simulink model "S1File_JL2005MM"  (R2017a)
settings: Solver=VariableStepAuto  StartTime=0.0  StopTime=96  RelTol=1e-3
libraries: cstblocks x2
settings Model: Creator=ac8227  LastModifiedBy=ac8227

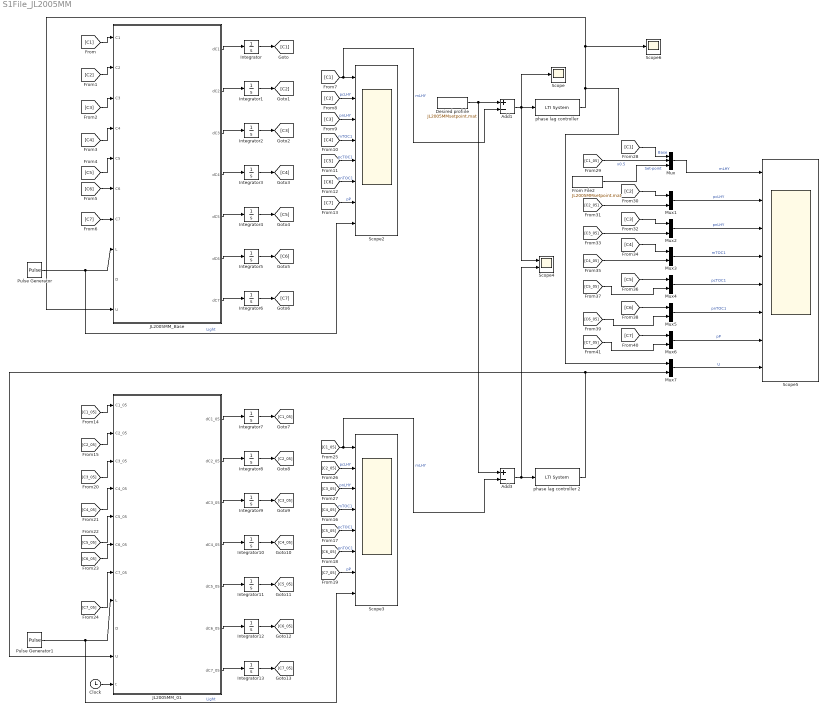
== system S1File_JL2005MM ==
  Add1 : Sum  Inputs=+-
  Add3 : Sum  Inputs=+-
  Clock : Clock
  Desired profiile : FromFile  FileName=JL2005MMsetpoint.mat  SampleTime=0
  From File2 : FromFile  FileName=JL2005MMsetpoint.mat  SampleTime=0
  Integrator : Integrator  InitialCondition=2.3718
  Integrator1 : Integrator  InitialCondition=1.2970
  Integrator10 : Integrator  InitialCondition=0.0740
  Integrator11 : Integrator  InitialCondition=1.0775
  Integrator12 : Integrator  InitialCondition=1.3873
  Integrator13 : Integrator  InitialCondition=0.1463
  Integrator2 : Integrator  InitialCondition=0.6887
  Integrator3 : Integrator  InitialCondition=0.0740
  Integrator4 : Integrator  InitialCondition=1.0775
  Integrator5 : Integrator  InitialCondition=1.3873
  Integrator6 : Integrator  InitialCondition=0.1463
  Integrator7 : Integrator  InitialCondition=2.3718
  Integrator8 : Integrator  InitialCondition=1.2970
  Integrator9 : Integrator  InitialCondition=0.6887
  JL2005MM_01 : MATLAB Function  TreatAsAtomicUnit=on
  JL2005MM_Base : MATLAB Function  TreatAsAtomicUnit=on
  Mux : Mux  Inputs=3
  Mux{1..7} (7 alike) : Mux  Inputs=2
  Pulse Generator : DiscretePulseGenerator  PulseType=Time based  Period=24  PulseWidth=50
  Pulse Generator1 : DiscretePulseGenerator  PulseType=Time based  Period=24  PulseWidth=50
  Scope : Scope
  Scope2 : Scope  NumInputPorts=8
  Scope3 : Scope  NumInputPorts=8
  Scope4 : Scope  NumInputPorts=2
  Scope5 : Scope  NumInputPorts=8
  Scope6 : Scope
  phase lag controller : cstblocks/LTI System  sys=tf([0.9],[1 0.026])  IC=[]
  phase lag controller 2 : cstblocks/LTI System  sys=tf([0.9],[1 0.026])  IC=[]
  wires:
  JL2005MM_Base/1(dC1) -> Integrator/1
  JL2005MM_Base/2(dC2) -> Integrator1/1
  JL2005MM_Base/3(dC3) -> Integrator2/1
  JL2005MM_Base/4(dC4) -> Integrator3/1
  JL2005MM_Base/5(dC5) -> Integrator4/1
  JL2005MM_Base/6(dC6) -> Integrator5/1
  JL2005MM_Base/7(dC7) -> Integrator6/1
  [C1] -> JL2005MM_Base/1(C1)
  [C2] -> JL2005MM_Base/2(C2)
  Integrator2/1 -> [C3]
  [C3] -> JL2005MM_Base/3(C3)
  Integrator3/1 -> [C4]
  [C4] -> JL2005MM_Base/4(C4)
  Integrator4/1 -> [C5]
  [C5] -> JL2005MM_Base/5(C5)
  Integrator5/1 -> [C6]
  Integrator6/1 -> [C7]
  [C7] -> JL2005MM_Base/7(C7)
  Pulse Generator/1 -> Scope2/8, JL2005MM_Base/8(L)  "Light"
  [C2] -> Scope2/2  "pcLHY"
  [C3] -> Scope2/3  "pnLHY"
  [C4] -> Scope2/4  "mTOC1"
  [C5] -> Scope2/5  "pcTOC1"
  [C6] -> Scope2/6  "pnTOC1"
  [C7] -> Scope2/7  "pP"
  [C1] -> Add1/2, Scope2/1  "mLHY"
  Integrator1/1 -> [C2]
  Add1/1 -> Scope4/1, Scope/1, phase lag controller/1
  [C1_05] -> JL2005MM_01/1(C1_05)
  [C1_05] -> Add3/2, Scope3/1  "mLHY"
  [C6_05] -> Scope3/6  "pnTOC1"
  [C3_05] -> Scope3/3  "pnLHY"
  JL2005MM_01/2(dC2_05) -> Integrator8/1
  [C4_05] -> Scope3/4  "mTOC1"
  [C5_05] -> Scope3/5  "pcTOC1"
  [C3_05] -> JL2005MM_01/3(C3_05)
  Integrator11/1 -> [C5_05]
  [C7_05] -> Scope3/7  "pP"
  [C2_05] -> Scope3/2  "pcLHY"
  [C4_05] -> JL2005MM_01/4(C4_05)
  JL2005MM_01/3(dC3_05) -> Integrator9/1
  JL2005MM_01/4(dC4_05) -> Integrator10/1
  Integrator13/1 -> [C7_05]
  Pulse Generator1/1 -> Scope3/8, JL2005MM_01/8(L)  "Light"
  [C5_05] -> JL2005MM_01/5(C5_05)
  Desired profiile/1 -> Add3/1, Add1/1
  Integrator10/1 -> [C4_05]
  JL2005MM_01/5(dC5_05) -> Integrator11/1
  [C2_05] -> JL2005MM_01/2(C2_05)
  Integrator9/1 -> [C3_05]
  JL2005MM_01/7(dC7_05) -> Integrator13/1
  JL2005MM_01/6(dC6_05) -> Integrator12/1
  Integrator12/1 -> [C6_05]
  [C6_05] -> JL2005MM_01/6(C6_05)
  [C7_05] -> JL2005MM_01/7(C7_05)
  Add3/1 -> Scope4/2, phase lag controller 2/1
  JL2005MM_01/1(dC1_05) -> Integrator7/1
  Integrator8/1 -> [C2_05]
  Integrator7/1 -> [C1_05]
  Mux7/1 -> Scope5/8  "U"
  Mux6/1 -> Scope5/7  "pP"
  Mux5/1 -> Scope5/6  "pnTOC1"
  Mux4/1 -> Scope5/5  "pcTOC1"
  Mux3/1 -> Scope5/4  "mTOC1"
  Mux2/1 -> Scope5/3  "pnLHY"
  Mux1/1 -> Scope5/2  "pcLHY"
  Mux/1 -> Scope5/1  "mLHY"
  [C2] -> Mux1/1
  [C2_05] -> Mux1/2
  [C3] -> Mux2/1
  [C3_05] -> Mux2/2
  [C4] -> Mux3/1
  [C4_05] -> Mux3/2
  [C5] -> Mux4/1
  [C5_05] -> Mux4/2
  [C6] -> Mux5/1
  [C6_05] -> Mux5/2
  [C7] -> Mux6/1
  [C7_05] -> Mux6/2
  [C1] -> Mux/1  "Base"
  [C1_05] -> Mux/2  "x0.5"
  From File2/1 -> Mux/3  "Set-point"
  [C6] -> JL2005MM_Base/6(C6)
  Integrator/1 -> [C1]
  phase lag controller/1 -> JL2005MM_Base/10(U), Scope6/1, Mux7/1
  phase lag controller 2/1 -> JL2005MM_01/10(U), Mux7/2
  Clock/1 -> JL2005MM_01/11(t)

== matlab function S1File_JL2005MM/JL2005MM_01 ==
  data: C1_05 input; dC1_05 output; C2_05 input; C3_05 input; C4_05 input; C5_05 input; C6_05 input; C7_05 input; L input; D input; dC2_05 output; dC3_05 output; dC4_05 output; dC5_05 output; dC6_05 output; dC7_05 output; U input; t input
function [dC1_05,dC2_05,dC3_05,dC4_05,dC5_05,dC6_05,dC7_05] = fcn(C1_05,C2_05,C3_05,C4_05,C5_05,C6_05,C7_05,L,D,U,t)

% Base level from Locke et al (2005) (MSE = 0.0627)
% prmLHY = [2.9741,16.9711,3.03510,9.3383,1.3294];
% prpcLHY = [4.9753,1.4563,0.8421,16.9058,0.8085];
% prpnLHY = [1.4563,0.8421,1.0214,0.1445];
% prmTOC1 = [0.1943,0.386,1.6859,0.2089];
% prpcTOC1 = [1.2947,0.0451,0.0018,0.4212,0.3187];
% prpnTOC1 = [0.0451,0.0018,0.0484,0.3505];
% prpP = [0.5,1.2,1.2,1];

% % Range of ~50 (MSE = 0.0057)
% prmLHY = [21.3829,3012.5858,97.1058,5740.9196,236.5913];
% prpcLHY = [5.1031,1.4973,1.5443,12.5909,0.3945];
% prpnLHY = [1.3618,0.60595,1.077,0.14356];
% prmTOC1 = [0.18959,0.42567,1.318,0.16526];
% prpcTOC1 = [1.2337,0.060339,0.0015998,0.35605,0.28326];
% prpnTOC1 = [0.045907,0.0017763,0.051637,0.40508];
% prpP = [0.45461,1.3044,1.626,0.67406];

% % Range of ~5 (MSE = 0.0066)
% prmLHY = [4.9338,25.8016,7.5373,58.7133,23.9218];
% prpcLHY = [4.8737,1.5378,0.93,16.2214,0.79457];
% prpnLHY = [1.3227,0.66914,0.94196,0.14577];
% prmTOC1 = [0.19031,0.37317,1.6321,0.21069];
% prpcTOC1 = [1.2674,0.045078,0.0018001,0.40754,0.29276];
% prpnTOC1 = [0.052677,0.0019858,0.056386,0.34943];
% prpP = [0.49324,1.2967,1.3816,1.066];

% % Range of ~0.5 (MSE = 0.0098)
% prmLHY = [1.6448,8.0011,0.63969,7.4748,0.6331];
% prpcLHY = [4.9944,1.3862,0.81083,16.3075,0.78208];
% prpnLHY = [1.5034,0.86568,1.0342,0.14472];
% prmTOC1 = [0.19694,0.35647,1.7854,0.19509];
% prpcTOC1 = [1.3478,0.04766,0.0018121,0.45754,0.31987];
% prpnTOC1 = [0.046707,0.001828,0.04697,0.3529];
% prpP = [0.50756,1.2094,1.2179,1.0118];

% % Range of ~0.05 (MSE = 0.0120)
% prmLHY = [5.7251,49.4649,0.078852,50.0593,0.11913];
% prpcLHY = [4.2229,1.5837,0.69777,15.801,0.90748];
% prpnLHY = [1.417,0.71977,0.93951,0.18241];
% prmTOC1 = [0.20527,0.3205,1.8736,0.1661];
% prpcTOC1 = [1.167,0.044472,0.0019508,0.38933,0.35667];
% prpnTOC1 = [0.048896,0.0022092,0.046747,0.2];
% prpP = [0.49541,1.38,1.4587,1.3033];

% % Range of ~0.005 (MSE = 0.0059)
% prmLHY = [4.0509,395.7813,0.0091778,395.8624,0.011849];
% prpcLHY = [5.392,1.3208,0.72844,19.4772,0.9734];
% prpnLHY = [1.3442,0.68392,0.9111,0.083128];
% prmTOC1 = [0.20498,0.4079,1.5483,0.19114];
% prpcTOC1 = [1.3518,0.048622,0.0025294,0.47169,0.43037];
% prpnTOC1 = [0.046706,0.0014573,0.049783,0.26696];
% prpP = [0.54185,1.2369,1.1099,1.5001];

%% New Set
% % Base level from Locke et al (2005) (MSE = 0.0627)
% prmLHY = [2.9741,16.9711,3.03510,9.3383,1.3294];
% prpcLHY = [4.9753,1.4563,0.8421,16.9058,0.8085];
% prpnLHY = [1.4563,0.8421,1.0214,0.1445];
% prmTOC1 = [0.1943,0.386,1.6859,0.2089];
% prpcTOC1 = [1.2947,0.0451,0.0018,0.4212,0.3187];
% prpnTOC1 = [0.0451,0.0018,0.0484,0.3505];
% prpP = [0.5,1.2,1.2,1];

% % Range of ~100 (MSE = 0.0057)
% prmLHY = [21.3829,3012.5858,97.1058,5740.9196,236.5913];
% prpcLHY = [5.1031,1.4973,1.5443,12.5909,0.3945];
% prpnLHY = [1.3618,0.60595,1.077,0.14356];
% prmTOC1 = [0.18959,0.42567,1.318,0.16526];
% prpcTOC1 = [1.2337,0.060339,0.0015998,0.35605,0.28326];
% prpnTOC1 = [0.045907,0.0017763,0.051637,0.40508];
% prpP = [0.45461,1.3044,1.626,0.67406];

% prmLHY = [51.4729,1228.3399,97.1058,3338.1188,325.5026];

% % Range of ~10 (MSE = 0.0066)
% prmLHY = [4.9338,25.8016,7.5373,58.7133,23.9218];
% prpcLHY = [4.8737,1.5378,0.93,16.2214,0.79457];
% prpnLHY = [1.3227,0.66914,0.94196,0.14577];
% prmTOC1 = [0.19031,0.37317,1.6321,0.21069];
% prpcTOC1 = [1.2674,0.045078,0.0018001,0.40754,0.29276];
% prpnTOC1 = [0.052677,0.0019858,0.056386,0.34943];
% prpP = [0.49324,1.2967,1.3816,1.066];

% % Range of ~0.1 (MSE = 0.0098)
% prmLHY = [1.6448,8.0011,0.63969,7.4748,0.6331];
% prpcLHY = [4.9944,1.3862,0.81083,16.3075,0.78208];
% prpnLHY = [1.5034,0.86568,1.0342,0.14472];
% prmTOC1 = [0.19694,0.35647,1.7854,0.19509];
% prpcTOC1 = [1.3478,0.04766,0.0018121,0.45754,0.31987];
% prpnTOC1 = [0.046707,0.001828,0.04697,0.3529];
% prpP = [0.50756,1.2094,1.2179,1.0118];

% % Range of ~0.01 (MSE = 0.0120)
% prmLHY = [5.7251,49.4649,0.078852,50.0593,0.11913];
% prpcLHY = [4.2229,1.5837,0.69777,15.801,0.90748];
% prpnLHY = [1.417,0.71977,0.93951,0.18241];
% prmTOC1 = [0.20527,0.3205,1.8736,0.1661];
% prpcTOC1 = [1.167,0.044472,0.0019508,0.38933,0.35667];
% prpnTOC1 = [0.048896,0.0022092,0.046747,0.2];
% prpP = [0.49541,1.38,1.4587,1.3033];

% % Range of ~0.001 (MSE = 0.0120)
prmLHY = [4.0509,395.7813,0.0091778,395.8624,0.011849];
prpcLHY = [5.392,1.3208,0.72844,19.4772,0.9734];
prpnLHY = [1.3442,0.68392,0.9111,0.083128];
prmTOC1 = [0.20498,0.4079,1.5483,0.19114];
prpcTOC1 = [1.3518,0.048622,0.0025294,0.47169,0.43037];
prpnTOC1 = [0.046706,0.0014573,0.049783,0.26696];
prpP = [0.54185,1.2369,1.1099,1.5001];

% Control problem: Suppose to due mutation, pnTOC1 is not producing, the
% controller will exert control action that mimic pnTOC1 for restore the
% overall circadian rhythm.

%% Optimisation
theta = [prmLHY prpcLHY prpnLHY prmTOC1 prpcTOC1 prpnTOC1 prpP];

% NOTE: Slight oscillation can avoid saturation of the control signal.

% LHY mRNA
dC1_05 = theta(1)*C7_05*L + (theta(2)*(0*C6_05 + 1*U))/(theta(3) + (0*C6_05 + 1*U)) - (theta(4)*C1_05)/(theta(5) + C1_05);
% dC1_05 = theta(1)*C7_05*L + (0*0.45*sin(2*pi/24*t) + 392.95) - (theta(4)*C1_05)/(theta(5) + C1_05);

% LHY protein cytosol
dC2_05 = theta(6)*C1_05 - theta(7)*C2_05 + theta(8)*C3_05 - (theta(9)*C2_05)/(theta(10) + C2_05);

% LHY protein nucleus
dC3_05 = theta(11)*C2_05 - theta(12)*C3_05 - (theta(13)*C3_05)/(theta(14) + C3_05);

% TOC1 mRNA
dC4_05 = theta(15)/(theta(16)^2 + C3_05^2) - (theta(17)*C4_05)/(theta(18) + C4_05);

% TOC1 protein cytosol
dC5_05 = theta(19)*C4_05 - theta(20)*C5_05 + theta(21)*C6_05 - (theta(22)*C5_05)/(theta(23) + C5_05);

% TOC1 protein nucleus
dC6_05 = theta(24)*C5_05 - theta(25)*C6_05 - (theta(26)*C6_05)/(theta(27) + C6_05)  + 0*D;

% Protein P
dC7_05 = (1 - L)*theta(28) - (theta(29)*C7_05)/(theta(30) + C7_05) - theta(31)*L*C7_05;

== matlab function S1File_JL2005MM/JL2005MM_Base ==
  data: C1 input; dC1 output; C2 input; C3 input; C4 input; C5 input; C6 input; C7 input; L input; D input; dC2 output; dC3 output; dC4 output; dC5 output; dC6 output; dC7 output; U input
function [dC1,dC2,dC3,dC4,dC5,dC6,dC7] = fcn(C1,C2,C3,C4,C5,C6,C7,L,D,U)

% Base level from Locke et al (2005) (MSE = 0.0627)
prmLHY = [2.9741,16.9711,3.03510,9.3383,1.3294];
prpcLHY = [4.9753,1.4563,0.8421,16.9058,0.8085];
prpnLHY = [1.4563,0.8421,1.0214,0.1445];
prmTOC1 = [0.1943,0.386,1.6859,0.2089];
prpcTOC1 = [1.2947,0.0451,0.0018,0.4212,0.3187];
prpnTOC1 = [0.0451,0.0018,0.0484,0.3505];
prpP = [0.5,1.2,1.2,1];

% Range of ~50 (MSE = 0.0057)
% prmLHY = [21.3829,3012.5858,97.1058,5740.9196,236.5913];
% prpcLHY = [5.1031,1.4973,1.5443,12.5909,0.3945];
% prpnLHY = [1.3618,0.60595,1.077,0.14356];
% prmTOC1 = [0.18959,0.42567,1.318,0.16526];
% prpcTOC1 = [1.2337,0.060339,0.0015998,0.35605,0.28326];
% prpnTOC1 = [0.045907,0.0017763,0.051637,0.40508];
% prpP = [0.45461,1.3044,1.626,0.67406];

% % Range of ~5 (MSE = 0.0066)
% prmLHY = [4.9338,25.8016,7.5373,58.7133,23.9218];
% prpcLHY = [4.8737,1.5378,0.93,16.2214,0.79457];
% prpnLHY = [1.3227,0.66914,0.94196,0.14577];
% prmTOC1 = [0.19031,0.37317,1.6321,0.21069];
% prpcTOC1 = [1.2674,0.045078,0.0018001,0.40754,0.29276];
% prpnTOC1 = [0.052677,0.0019858,0.056386,0.34943];
% prpP = [0.49324,1.2967,1.3816,1.066];

% % Range of ~0.5 (MSE = 0.0098)
% prmLHY = [1.6448,8.0011,0.63969,7.4748,0.6331];
% prpcLHY = [4.9944,1.3862,0.81083,16.3075,0.78208];
% prpnLHY = [1.5034,0.86568,1.0342,0.14472];
% prmTOC1 = [0.19694,0.35647,1.7854,0.19509];
% prpcTOC1 = [1.3478,0.04766,0.0018121,0.45754,0.31987];
% prpnTOC1 = [0.046707,0.001828,0.04697,0.3529];
% prpP = [0.50756,1.2094,1.2179,1.0118];

% % Range of ~0.05 (MSE = 0.0120)
% prmLHY = [5.7251,49.4649,0.078852,50.0593,0.11913];
% prpcLHY = [4.2229,1.5837,0.69777,15.801,0.90748];
% prpnLHY = [1.417,0.71977,0.93951,0.18241];
% prmTOC1 = [0.20527,0.3205,1.8736,0.1661];
% prpcTOC1 = [1.167,0.044472,0.0019508,0.38933,0.35667];
% prpnTOC1 = [0.048896,0.0022092,0.046747,0.2];
% prpP = [0.49541,1.38,1.4587,1.3033];

% Control problem: Suppose to due mutation, pnTOC1 is not producing, the
% controller will exert control action that mimic pnTOC1 for restore the
% overall circadian rhythm.

%% Optimisation
theta = [prmLHY prpcLHY prpnLHY prmTOC1 prpcTOC1 prpnTOC1 prpP];

% LHY mRNA
dC1 = theta(1)*C7*L + (theta(2)*(0*C6 + 1*U))/(theta(3) + (0*C6 + 1*U)) - (theta(4)*C1)/(theta(5) + C1);

% LHY protein cytosol
dC2 = theta(6)*C1 - theta(7)*C2 + theta(8)*C3 - (theta(9)*C2)/(theta(10) + C2);

% LHY protein nucleus
dC3 = theta(11)*C2 - theta(12)*C3 - (theta(13)*C3)/(theta(14) + C3);

% TOC1 mRNA
dC4 = theta(15)/(theta(16)^2 + C3^2) - (theta(17)*C4)/(theta(18) + C4);

% TOC1 protein cytosol
dC5 = theta(19)*C4 - theta(20)*C5 + theta(21)*C6 - (theta(22)*C5)/(theta(23) + C5);

% TOC1 protein nucleus
dC6 = theta(24)*C5 - theta(25)*C6 - (theta(26)*C6)/(theta(27) + C6)  + 0*D;

% Protein P
dC7 = (1 - L)*theta(28) - (theta(29)*C7)/(theta(30) + C7) - theta(31)*L*C7;
